simulink model "motor_control"  (R2024b)
settings: Solver=FixedStepDiscrete  StartTime=0.0  StopTime=inf  FixedStep=0.001  RelTol=1e-3  EnableMultiTasking=on
InitFcn:
  | % Check we are building from the correct Build folder
  | expectedDir = 'Motor_Control\Build';
  | currentDir  = pwd;
  | 
  | if ~contains(currentDir, expectedDir)
  |     error(['Wrong folder! You must run from the Build folder.' ...
  |            '\nCurrent: %s' ...
  |            '\nExpected path to contain: %s'], ...
  |            currentDir, expectedDir);
  | end
  | 
  | % Load all signals and parameters
  | loadall();
undefined symbols (not defined in the file): BEnableLedBlink
libraries: simulink x6, stm32f4xxblockslib x2, myLib x1
settings Model: STM32="{\"DigitalPortWrite\":{\"ID\":\"motor_control:4\"},\"DigitalPortRead\":{\"ID\":\"motor_control:237\"}}"  SimulationMode=external  ExtModeEnableFloating=off  Creator=sakee  LastModifiedBy=sakee
settings SolverCC: PositivePriorityOrder=on  AutoInsertRateTranBlk=on
settings OptimizationCC: EnhancedBackFolding=on  PassReuseOutputArgsAs=Individual arguments  ZeroExternalMemoryAtStartup=off  ZeroInternalMemoryAtStartup=off  MaxStackSize=512  OptimizeBlockOrder=speed  DifferentSizesBufferReuse=on  OptimizationCustomize=off  EfficientTunableParamExpr=on
settings DebuggingCC: MultiTaskDSMMsg=warning  ParameterTunabilityLossMsg=error
settings HardwareCC: ProdBitPerPointer=32  ProdBitPerSizeT=32  ProdBitPerPtrDiffT=32  ProdLargestAtomicInteger=Long  ProdLargestAtomicFloat=Double  ProdWordSize=32  ProdLongLongMode=on  ProdHWDeviceType=ARM Compatible->ARM Cortex-M
settings SFSimCC: MATLABDynamicMemAlloc=off
settings RTWCC: Description=Embedded Coder  SystemTargetFile=ert.tlc  HardwareBoard=STM32G4xx Based  TLCOptions="-aInlineSetEventsForThisBaseRateFcn=TLC_FALSE -aSuppressMultiTaskScheduler=TLC_FALSE    -aRateBasedStepFcn=0"  TemplateMakefile=ert_default_tmf  Toolchain=GNU Tools for ARM Embedded Processors
settings CodeAppCC: ForceParamTrailComments=on  IgnoreCustomStorageClasses=off  OperatorAnnotations=on  SimulinkDataObjDesc=on  SFDataObjDesc=on  InsertBlockDesc=on
settings ERTTargetCC: TargetLangStandard=C99 (ISO)  CodeReplacementLibrary=ARM Cortex-M  ExtModeTransport=3  ExtModeStaticAlloc=on  ExtModeStaticAllocSize=2048  ExtModeMexFile=ext_xcp  ExtModeIntrfLevel=Level2 - Open  InlinedParameterPlacement=Hierarchical

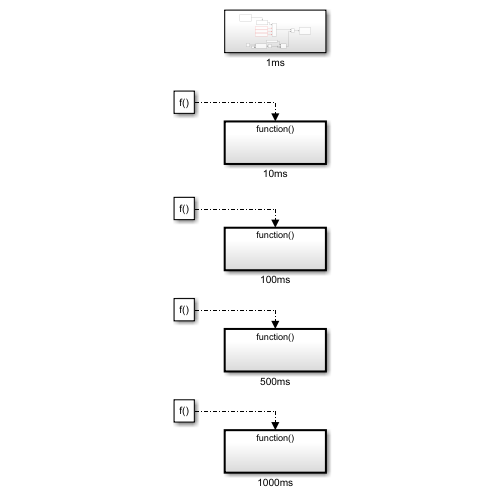
[thumbnail: Simulink's stored preview of the top-level diagram]
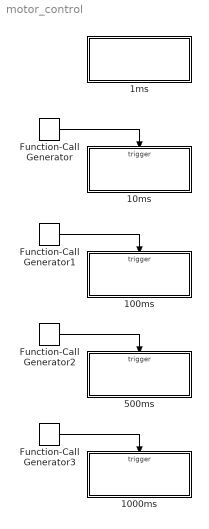
== system motor_control ==
  1000ms : Subsystem  TreatAsAtomicUnit=on
  100ms : Subsystem  TreatAsAtomicUnit=on
  10ms : Subsystem  TreatAsAtomicUnit=on
  1ms : Subsystem
  500ms : Subsystem  TreatAsAtomicUnit=on
  Function-Call Generator : simulink/Ports & Subsystems/Function-Call Generator  sample_time=0.01  numberOfIterations=1  DisallowWideOutput=off
  Function-Call Generator1 : simulink/Ports & Subsystems/Function-Call Generator  sample_time=0.1  numberOfIterations=1  DisallowWideOutput=off
  Function-Call Generator2 : simulink/Ports & Subsystems/Function-Call Generator  sample_time=0.5  numberOfIterations=1  DisallowWideOutput=off
  Function-Call Generator3 : simulink/Ports & Subsystems/Function-Call Generator  sample_time=1  numberOfIterations=1  DisallowWideOutput=off
  wires:
  Function-Call Generator/1 -> 10ms/Trigger
  Function-Call Generator1/1 -> 100ms/Trigger
  Function-Call Generator2/1 -> 500ms/Trigger
  Function-Call Generator3/1 -> 1000ms/Trigger

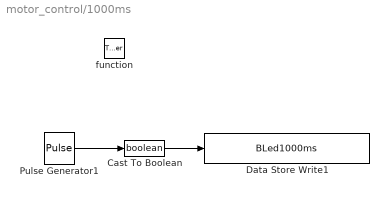
== system motor_control/1000ms ==
  function : TriggerPort  TriggerType=function-call  VariantControl=(inherit)
  Cast To Boolean : DataTypeConversion  OutDataTypeStr=boolean  SaturateOnIntegerOverflow=off  RndMeth=Floor
  Data Store Write1 : DataStoreWrite  DataStoreName=BLed1000ms  IndexOptions=Index vector (dialog)  Indices=1  OutputSizes=1
  Pulse Generator1 : DiscretePulseGenerator  SampleTime=-1
  wires:
  Pulse Generator1/1 -> Cast To Boolean/1
  Cast To Boolean/1 -> Data Store Write1/1

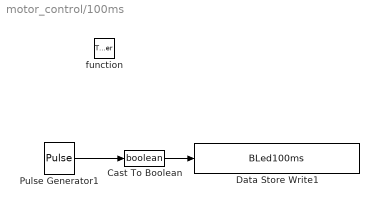
== system motor_control/100ms ==
  function : TriggerPort  TriggerType=function-call  VariantControl=(inherit)
  Cast To Boolean : DataTypeConversion  OutDataTypeStr=boolean  SaturateOnIntegerOverflow=off  RndMeth=Floor
  Data Store Write1 : DataStoreWrite  DataStoreName=BLed100ms  IndexOptions=Index vector (dialog)  Indices=1  OutputSizes=1
  Pulse Generator1 : DiscretePulseGenerator  SampleTime=-1
  wires:
  Cast To Boolean/1 -> Data Store Write1/1
  Pulse Generator1/1 -> Cast To Boolean/1

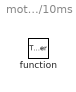
== system motor_control/10ms ==
  function : TriggerPort  TriggerType=function-call  VariantControl=(inherit)

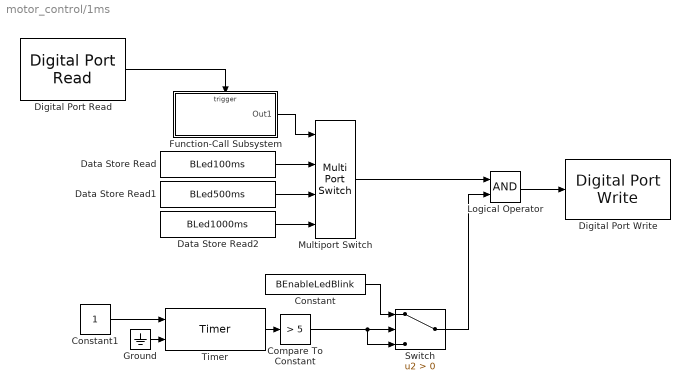
== system motor_control/1ms ==
  Compare To Constant : simulink/Logic and Bit Operations/Compare To Constant  relop=>  const=5  OutDataTypeStr=boolean
  Constant : Constant  Value=BEnableLedBlink
  Constant1 : Constant
  Data Store Read : DataStoreRead  DataStoreName=BLed100ms  IndexOptions=Index vector (dialog)  Indices=1  OutputSizes=1
  Data Store Read1 : DataStoreRead  DataStoreName=BLed500ms  IndexOptions=Index vector (dialog)  Indices=1  OutputSizes=1
  Data Store Read2 : DataStoreRead  DataStoreName=BLed1000ms  IndexOptions=Index vector (dialog)  Indices=1  OutputSizes=1
  Digital Port Read : stm32f4xxblockslib/Digital Port Read  PortName=GPIOC  PinNumber=10  ReadOperation=on  IOAsArray=on  SampleTime=-1  EnableSimPort=off  hoistedMaskSrc=ECSoC/ECSimCodegen/Digital Port Read
      settings: LibrarySourceBlock=stm32g4xxblockslib/Digital Port Read
  Digital Port Write : stm32f4xxblockslib/Digital Port Write  PortName=GPIOC  PinNumber=6  ReadOperation=off  IOAsArray=off  EnableSimPort=off  hoistedMaskSrc=ECSoC/ECSimCodegen/Digital Port Write
  Function-Call Subsystem : Subsystem  TreatAsAtomicUnit=on
  Ground : Ground
  Logical Operator : Logic  AllPortsSameDT=off  OutDataTypeStr=boolean
  Multiport Switch : MultiPortSwitch  DataPortOrder=Zero-based contiguous  zeroidx=on  SaturateOnIntegerOverflow=off  InputSameDT=off
  Switch : Switch  Criteria=u2 > Threshold  SaturateOnIntegerOverflow=off  InputSameDT=off
  Timer : myLib/Timer  tSampleTime=0.001
  wires:
  Function-Call Subsystem/1(Out1) -> Multiport Switch/1
  Multiport Switch/1 -> Logical Operator/1
  Logical Operator/1 -> Digital Port Write/1
  Data Store Read/1 -> Multiport Switch/2
  Data Store Read1/1 -> Multiport Switch/3
  Data Store Read2/1 -> Multiport Switch/4
  Digital Port Read/1 -> Function-Call Subsystem/Trigger
  Constant1/1 -> Timer/1
  Ground/1 -> Timer/2
  Timer/1 -> Compare To Constant/1
  Compare To Constant/1 -> Switch/3, Switch/2
  Constant/1 -> Switch/1
  Switch/1 -> Logical Operator/2

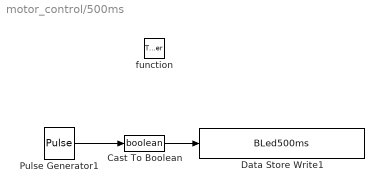
== system motor_control/500ms ==
  function : TriggerPort  TriggerType=function-call  VariantControl=(inherit)
  Cast To Boolean : DataTypeConversion  OutDataTypeStr=boolean  SaturateOnIntegerOverflow=off  RndMeth=Floor
  Data Store Write1 : DataStoreWrite  DataStoreName=BLed500ms  IndexOptions=Index vector (dialog)  Indices=1  OutputSizes=1
  Pulse Generator1 : DiscretePulseGenerator  SampleTime=-1
  wires:
  Pulse Generator1/1 -> Cast To Boolean/1
  Cast To Boolean/1 -> Data Store Write1/1

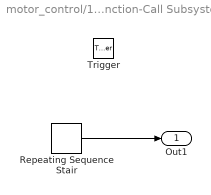
== system motor_control/1ms/Function-Call Subsystem ==
  Trigger : TriggerPort  VariantControl=(inherit)  PortDimensions=1
  Repeating Sequence Stair : simulink/Sources/Repeating Sequence Stair  OutValues=[1 2 0]  tsamp=-1  OutMin=[]  OutMax=[]  OutDataTypeStr=double  OutputDataTypeScalingMode=double  OutDataType=fixdt(0,8)  ConRadixGroup=Best Precision: Vector-wise  OutScaling=2^-12
  Out1 : Outport
  wires:
  Repeating Sequence Stair/1 -> Out1/1
